simulink model "EjemploPioneer"  (Simulink 8.4)
settings: Solver=FixedStepDiscrete  StartTime=0.0  StopTime=inf  FixedStep=0.01  RelTol=1e-3
settings Model: Creator=Usuario  LastModifiedBy=dds

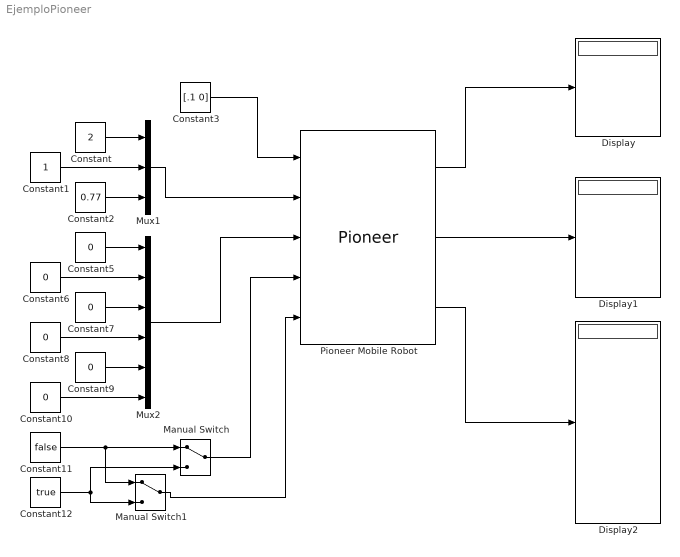
== system EjemploPioneer ==
  Constant : Constant  Value=2
  Constant1 : Constant
  Constant{5..10} (6 alike) : Constant  Value=0  OutDataTypeStr=int32
  Constant11 : Constant  Value=false
  Constant12 : Constant  Value=true
  Constant2 : Constant  Value=0.77
  Constant3 : Constant  Value=[.1 0]
  Display : Display
  Display1 : Display
  Display2 : Display
  Manual Switch : ManualSwitch
  Manual Switch1 : ManualSwitch
  Mux1 : Mux  Inputs=3
  Mux2 : Mux  Inputs=6
  Pioneer Mobile Robot : S-Function  FunctionName=Pioneer  Parameters=1  EnableBusSupport=off
      mask Display:
      | color('red')
      | port_label('input',1,'acciones')
      | port_label('input',2,'postura')
      | port_label('input',3,'parametros')
      | port_label('input',4,'parametrosSend')
      | port_label('input',5,'posturaSend')
      | color('blue')
      | port_label('output',1,'estado')
      | port_label('output',2,'parametros')
      | port_label('output',3,'laser')
  wires:
  Constant/1 -> Mux1/1
  Constant1/1 -> Mux1/2
  Constant2/1 -> Mux1/3
  Constant5/1 -> Mux2/1
  Constant6/1 -> Mux2/2
  Constant7/1 -> Mux2/3
  Constant8/1 -> Mux2/4
  Constant9/1 -> Mux2/5
  Constant10/1 -> Mux2/6
  Constant11/1 -> Manual Switch/1, Manual Switch1/1
  Constant12/1 -> Manual Switch/2, Manual Switch1/2
  Manual Switch/1 -> Pioneer Mobile Robot/4
  Manual Switch1/1 -> Pioneer Mobile Robot/5
  Mux1/1 -> Pioneer Mobile Robot/2
  Mux2/1 -> Pioneer Mobile Robot/3
  Pioneer Mobile Robot/2 -> Display1/1
  Pioneer Mobile Robot/1 -> Display/1
  Pioneer Mobile Robot/3 -> Display2/1
  Constant3/1 -> Pioneer Mobile Robot/1
